simulink model "zero_input_lqr"  (R2024a)
settings: Solver=VariableStepAuto  StartTime=0.0  StopTime=30  RelTol=1e-3
values from neighbouring files (symbols this model uses):
  A = [-1.7, -0.25, 0 ... (first row only)    [main.m]
  B = [7, 0 ... (first row only)    [main.m]
  x0 = [1 100 200]'    [main.m]
undefined symbols (not defined in the file or in its folder): K_own
settings Model: Creator=chint  LastModifiedBy=chint

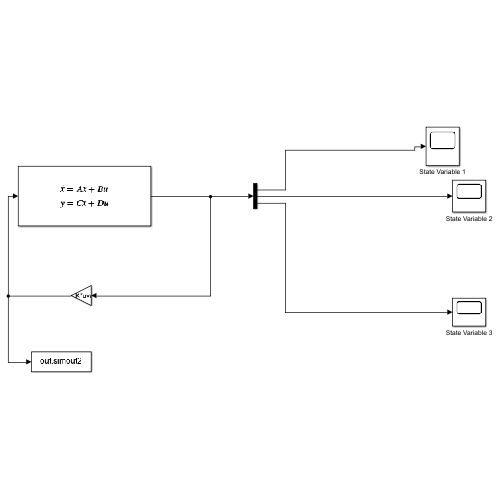
[thumbnail: Simulink's stored preview of the top-level diagram]
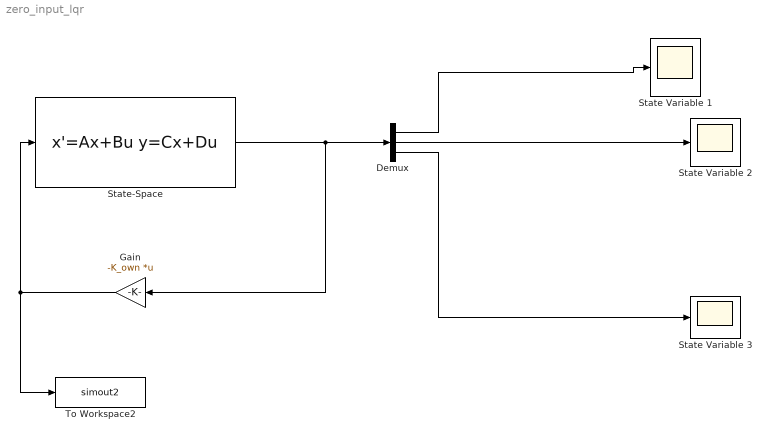
== system zero_input_lqr ==
  Demux : Demux  Outputs=3
  Gain : Gain  Gain=-K_own  Multiplication=Matrix(K*u) (u vector)
  State Variable 1 : Scope
  State Variable 2 : Scope
  State Variable 3 : Scope
  State-Space : StateSpace  A=A  B=B  C=eye(3)  D=[0 0; 0 0; 0 0]  InitialCondition=x0
  To Workspace2 : ToWorkspace  VariableName=simout2  SaveFormat=Timeseries  SampleTime=-1
  wires:
  Gain/1 -> To Workspace2/1, State-Space/1
  State-Space/1 -> Demux/1, Gain/1
  Demux/2 -> State Variable 2/1
  Demux/3 -> State Variable 3/1
  Demux/1 -> State Variable 1/1
